simulink model "ex5_StateChart"  (R2024a)
settings: Solver=FixedStepDiscrete  StartTime=0.0  StopTime=10.0  FixedStep=0.0001  RelTol=1e-3  EnableMultiTasking=on
settings Model: Creator=erfuu  LastModifiedBy=erfuu
settings SolverCC: AlgebraicLoopSolver=TrustRegion  AutoInsertRateTranBlk=on
settings DataIOCC: LimitDataPoints=on
settings OptimizationCC: DefaultParameterBehavior=Inlined  EnhancedBackFolding=on  PassReuseOutputArgsAs=Individual arguments  ZeroExternalMemoryAtStartup=off  ZeroInternalMemoryAtStartup=off  OptimizeBlockOrder=speed  DifferentSizesBufferReuse=on  OptimizationCustomize=off  EfficientTunableParamExpr=on
settings DebuggingCC: ParameterTunabilityLossMsg=error  UnconnectedInputMsg=warning  UnconnectedOutputMsg=warning  UnconnectedLineMsg=warning  AllowSymbolicDim=off  SFUnexpectedBacktrackingDiag=warning  SFNoUnconditionalDefaultTransitionDiag=warning  SFExecutionAtInitializationDiag=none  ArithmeticOperatorsInVariantConditions=warning
settings ModelReferenceCC: EnableRefExpFcnMdlSchedulingChecks=on
settings SFSimCC: SimUseLocalCustomCode=off  MATLABDynamicMemAlloc=off  CustomCodeUndefinedFunction=UseInterfaceOnly
settings RTWCC: Description=Embedded Coder  SystemTargetFile=ert.tlc  TemplateMakefile=ert_default_tmf  RTWUseLocalCustomCode=off  GPUComputeCapability=3.5  DLArmComputeVersion=19.05
settings CodeAppCC: ForceParamTrailComments=on  IgnoreCustomStorageClasses=off  OperatorAnnotations=on  SimulinkDataObjDesc=on  SFDataObjDesc=on  InsertBlockDesc=on
settings ERTTargetCC: GenerateSampleERTMain=on  InlinedParameterPlacement=NonHierarchical  ERTCustomFileTemplate=example_file_process.tlc
settings ConfigComp: CovMetricSettings=dw  CovSaveCumulativeToWorkspaceVar=on  CovSaveSingleToWorkspaceVar=on  CovExternalEMLEnable=off

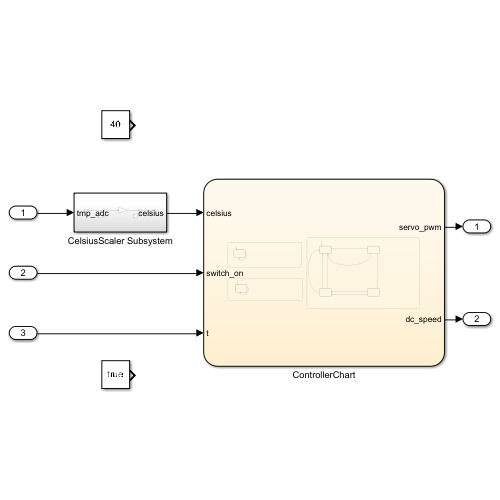
[thumbnail: Simulink's stored preview of the top-level diagram]
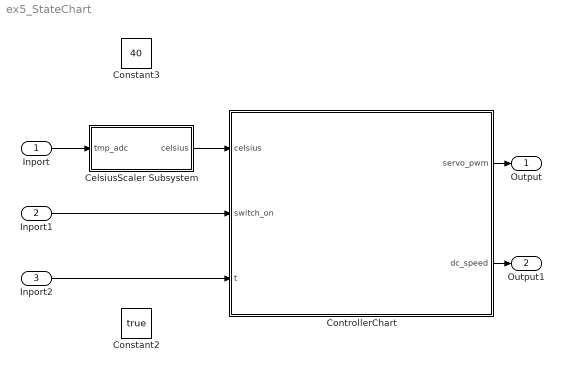
== system ex5_StateChart ==
  Inport : Inport
  Inport1 : Inport  Port=2
  Inport2 : Inport  Port=3
  CelsiusScaler Subsystem : Subsystem
  Constant2 : Constant  Value=true
  Constant3 : Constant  Value=40
  ControllerChart : Stateflow chart  TreatAsAtomicUnit=on
  Output : Outport
  Output1 : Outport  Port=2
  wires:
  ControllerChart/1(servo_pwm) -> Output/1
  ControllerChart/2(dc_speed) -> Output1/1
  Inport/1 -> CelsiusScaler Subsystem/1(tmp_adc)
  CelsiusScaler Subsystem/1(celsius) -> ControllerChart/1(celsius)
  Inport1/1 -> ControllerChart/2(switch_on)
  Inport2/1 -> ControllerChart/3(t)

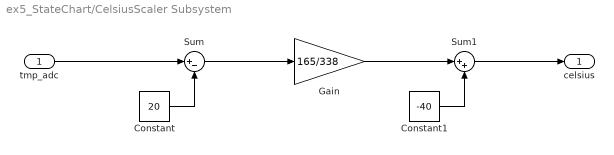
== system ex5_StateChart/CelsiusScaler Subsystem ==
  tmp_adc : Inport
  Constant : Constant  Value=20
  Constant1 : Constant  Value=-40
  Gain : Gain  Gain=165/338
  Sum : Sum  Inputs=|+-
  Sum1 : Sum  Inputs=|++
  celsius : Outport
  wires:
  Constant/1 -> Sum/2
  tmp_adc/1 -> Sum/1
  Constant1/1 -> Sum1/2
  Gain/1 -> Sum1/1
  Sum1/1 -> celsius/1
  Sum/1 -> Gain/1

== stateflow chart ex5_StateChart/ControllerChart ==
  state Servo_Motor [parallel]
    settings: executionOrder=3
    state Pulse_High
    state Pulse_Down
    state Check_Direction
    state Check_Mode
    (default) -> Pulse_High : {servo_pwm = 1}
    Pulse_High -> Pulse_Down : [rem(t, servo_pw) == 0]{servo_pwm = 0}
    Check_Direction -> Pulse_High [order 3]
    Check_Direction -> Pulse_High [order 1] : [servo_pw >= SERVO_MAX_PW]{servo_dir = -1}
    Check_Direction -> Pulse_High [order 2] : [servo_pw <= SERVO_MIN_PW]{servo_dir = 1}
    Pulse_Down -> Pulse_High [order 2] : [rem(t, SERVO_PERIOD) == 0 && rem(t, JUMP * SERVO_PERIOD ) ~= 0]{servo_pwm = 1}
    Pulse_Down -> Check_Mode [order 1] : [rem(t, SERVO_PERIOD) == 0 && rem(t, JUMP * SERVO_PERIOD) == 0]{servo_pwm = 1}
    Check_Mode -> Check_Direction [order 2] : [fast_mode == 1]{servo_pw = servo_pw + JUMP * servo_dir * 2 * (SERVO_MAX_PW - SERVO_MIN_PW) / (FAST_MODE_DURATION / SERVO_PERIOD)}
    Check_Mode -> Check_Direction [order 1] : [fast_mode == 1]{servo_pw = servo_pw + JUMP * servo_dir * 2 * (SERVO_MAX_PW - SERVO_MIN_PW) / (SLOW_MODE_DURATION / SERVO_PERIOD)}
  state DC_Motor [parallel]
    settings: executionOrder=1
    state s2
    (default) -> s2
    s2 -> s2 : [rem(t,SENSOR_PERIOD)  == 0]{dc_speed = (celsius - 20) * DC_MAX_SPEED / (DC_MAX_RPM / 60) }
  state Switch [parallel]
    settings: executionOrder=2
    state s3
    (default) -> s3
    s3 -> s3 : [rem(t,SWITCH_PERIOD) == 0]{fast_mode = switch_on}
  data: celsius input; switch_on input; servo_pwm output =0; dc_speed output =0; SERVO_PERIOD constant double =20000; SERVO_MAX_PW constant double =2000; SERVO_MIN_PW constant double =1000; SLOW_MODE_DURATION constant double =10000000; FAST_MODE_DURATION constant double =5000000; SWITCH_PERIOD constant double =100000; SENSOR_PERIOD constant double =1000000; fast_mode local =0; servo_pw local =1000; servo_dir local =1; DC_MAX_SPEED constant double =255; DC_MAX_RPM local =16530; JUMP constant double =25; t input double =0
